simulink model "ev"  (R2021a)
settings: Solver=ode4  StartTime=0  StopTime=1082  FixedStep=sim_dt  RelTol=1e-3
model workspace (MAT data in the model file):
  T_eff_bp = [-270; -210; -150; -90; -30; 30; 90; 150; 210; 270]
  T_eff_bp_2 = [-270; -210; -150; -90; -30; 30; 90; 150; 210; 270]
  losses_table = [108927.107777 7820.2782368 7820.17609997 7820.2782368 7820.2782368 7820.2782368 7820.2782368 7820.26172359 7820.2782368 9345.38006027 108927.107777 7820.2782368 ... (100 elements, 10x10)]
  losses_table_2 = [108927.107777 7820.2782368 7820.17609997 7820.2782368 7820.2782368 7820.2782368 7820.2782368 7820.26172359 7820.2782368 9345.38006027 108927.107777 7820.2782368 ... (100 elements, 10x10)]
  w_eff_bp = [0; 888.888888889; 1777.77777778; 2666.66666667; 3555.55555556; 4444.44444444; 5333.33333333; 6222.22222222; 7111.11111111; 8000]
  w_eff_bp_2 = [0; 888.888888889; 1777.77777778; 2666.66666667; 3555.55555556; 4444.44444444; 5333.33333333; 6222.22222222; 7111.11111111; 8000]
undefined symbols (not defined in the file): Af, alpha, Bt, C, C_fa, C_free, C_sa_bat, C_sa_uc, Cd, Cmax, Continuous, Crr, DoD, effi, etaFD, etaG, FD, G, gear, Iucmax, m, M1m, M2m, Max, npar, npar_free, npara, nparf, nparfa, nparsa_bat, nparsa_UC, nser, nser_free, nserfa, nsersa_bat, nsersa_UC, Qbat, regenmax, Ri_BP, RL, ro, Rsc, Rsc_A, Rsc_F, Rsc_sa_bat, Rsc_sa_uc, rw, sim_dt, SOC_BP, SoCbatmax, SoCbatmin, SoCucmax, SoCucmin, speed, torque, VinBat, Voc_BP, Vuc, Vuc_fa, Vuc_free ... (+2)
libraries: autolibshared x41, simulink x26, autolibdcdc x13, autolibdatasheetbattery x7, autolibmappedmotor x6, fl_lib x3, nesl_utility x3, spsSupercapacitorLib x3, pid_lib x1
(part 9 of 18)

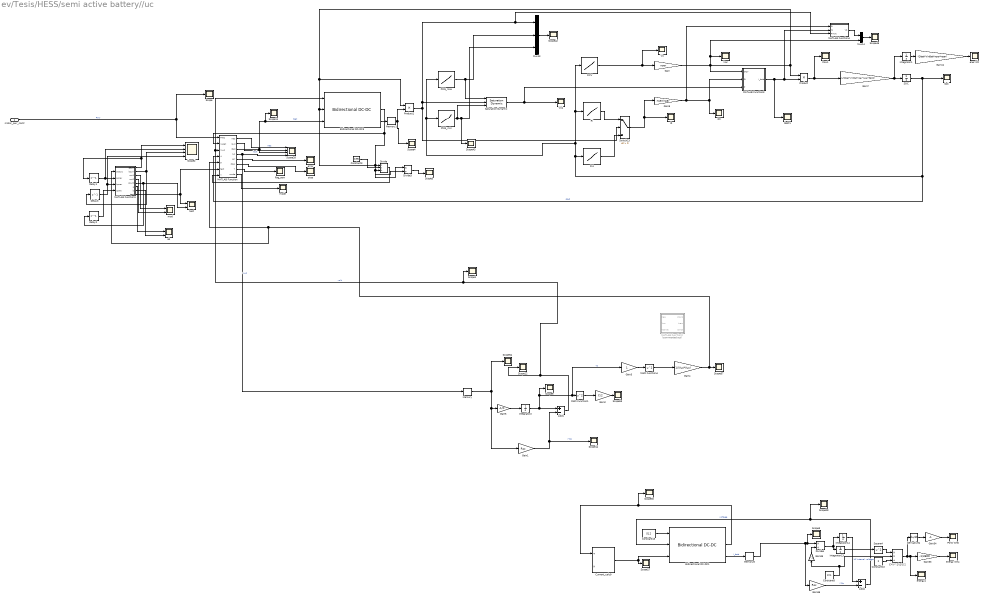
== system ev/Tesis/HESS/semi active battery//uc ==
  motor_pwr_contr : Inport
  Add1 : Sum  Inputs=+-
  Add4 : Sum  Inputs=+-
  Bidirectional DC-DC1 : autolibdcdc/Bidirectional DC-DC  Tc=1/1000  Vinit=51.2  Plimit=100000  param_loss=Single efficiency measurement  eff=95  v_loss_bp=[0 200 400 600 800 1000]  i_loss_bp=[0 25 50 75 100]  losses_table=[100 100 100 100 100;100 150 200 250 300;100 200 300 400 500;100 250 400 550 700;100 300 500 700 900;100 350 600 850 1100]  v_eff_bp=[200 400 600 800 1000]  i_eff_bp=[25 50 75 100]  efficiency_table=[96.2 98.1 98.7 99;98.1 99 99.4 99.5;98.7 99.4 99.6 99.7;99 99.5 99.7 99.8;99.2 99.6 99.7 99.8]  x_v_bp=[-1000 -800 -600 -400 -200 200 400 600 800 1000]  x_i_bp=[-100 -75 -50 -25 25 50 75 100]  x_losses_mat=[200.400801603196 225.67703109328 200.803212851408 201.612903225806 199.999999999997 200 225 200;160.320641282556 180.541624874624 201.005025125625 202.020202020203 200 200 180 160;180.541624874624 180.722891566267 181.086519114686 197.568389057748 194.999999999999 179.999999999997 180 180;201.005025125625 181.086519114686 202.020202020203 193.67991845056 190 200 179.999999999997 200;202.020202020203 197.568389057748 193.67991845056 197.505197505197 190 190 194.999999999999 200;200 194.999999999999 190 190 197.505197505197 193.67991845056 197.568389057748 202.020202020203;200 179.999999999997 200 190 193.67991845056 202.020202020203 181.086519114686 201.005025125625;180 180 179.999999999997 194.999999999999 197.568389057748 181.086519114686 180.722891566267 180.541624874624;160 180 200 200 202.020202020203 201.005025125625 180.541624874624 160.320641282556;200 225 200 199.999999999997 201.612903225806 200.803212851408 225.67703109328 200.400801603196]  RefBlkName='autolibdcdc/Bidirectional DC-DC'
      settings: SourceProductBaseCode=PW
  Bidirectional DC-DC3 : autolibdcdc/Bidirectional DC-DC  Tc=1/1000  Vinit=48  Plimit=100000  param_loss=Single efficiency measurement  eff=95  v_loss_bp=[0 200 400 600 800 1000]  i_loss_bp=[0 25 50 75 100]  losses_table=[100 100 100 100 100;100 150 200 250 300;100 200 300 400 500;100 250 400 550 700;100 300 500 700 900;100 350 600 850 1100]  v_eff_bp=[200 400 600 800 1000]  i_eff_bp=[25 50 75 100]  efficiency_table=[96.2 98.1 98.7 99;98.1 99 99.4 99.5;98.7 99.4 99.6 99.7;99 99.5 99.7 99.8;99.2 99.6 99.7 99.8]  x_v_bp=[-1000 -800 -600 -400 -200 200 400 600 800 1000]  x_i_bp=[-100 -75 -50 -25 25 50 75 100]  x_losses_mat=[200.400801603196 225.67703109328 200.803212851408 201.612903225806 199.999999999997 200 225 200;160.320641282556 180.541624874624 201.005025125625 202.020202020203 200 200 180 160;180.541624874624 180.722891566267 181.086519114686 197.568389057748 194.999999999999 179.999999999997 180 180;201.005025125625 181.086519114686 202.020202020203 193.67991845056 190 200 179.999999999997 200;202.020202020203 197.568389057748 193.67991845056 197.505197505197 190 190 194.999999999999 200;200 194.999999999999 190 190 197.505197505197 193.67991845056 197.568389057748 202.020202020203;200 179.999999999997 200 190 193.67991845056 202.020202020203 181.086519114686 201.005025125625;180 180 179.999999999997 194.999999999999 197.568389057748 181.086519114686 180.722891566267 180.541624874624;160 180 200 200 202.020202020203 201.005025125625 180.541624874624 160.320641282556;200 225 200 199.999999999997 201.612903225806 200.803212851408 225.67703109328 200.400801603196]  RefBlkName='autolibdcdc/Bidirectional DC-DC'
      settings: SourceProductBaseCode=PW
  C*(V^2)/2(1)2 : Product  Inputs=**/
  Constant10 : Constant  Value=2
  Constant13 : Constant  Value=51.2
  Constant3 : Constant  Value=0.95
  Constant8 : Constant  Value=C*1
  Current_calc9 : Product  Inputs=/*
  Delay1 : Delay  DelayLength=1  InitialCondition=1
  Delay2 : Delay  DelayLength=1  InitialCondition=1
  Delay3 : Delay  DelayLength=1  InitialCondition=1
  Derivative4 : Derivative
  Divide : Product  Inputs=**/
  Divide3 : Product  Inputs=*/
  Divide4 : Product  Inputs=*/
  Gain : Gain  Gain=nser
  Gain1 : Gain  Gain=Rsc
  Gain11 : Gain  Gain=(Qbat*VinBat*nser*npar)
  Gain2 : Gain  Gain=C/2
  Gain3 : Gain
  Gain33 : Gain  Gain=-1/3600
  Gain34 : Gain  Gain=-1
  Gain35 : Gain  Gain=-1
  Gain36 : Gain  Gain=Rsc
  Gain4 : Gain  Gain=1/(Vuc*Vuc)
  Gain5 : Gain  Gain=-1/C
  Gain6 : Gain  Gain=nser/npar
  Gain7 : Gain  Gain=1/(Qbat*VinBat*nser*npar*3600)
  Ibatt1 : Scope
  Integrator1 : Integrator
  Integrator13 : Integrator
  Integrator14 : Integrator  InitialCondition=Vuc*1
  Integrator2 : Integrator  InitialCondition=48  UpperSaturationLimit=Vuc  LowerSaturationLimit=Vuc*0
  MATLAB Function : MATLAB Function  TreatAsAtomicUnit=on
  MATLAB Function1 : MATLAB Function  TreatAsAtomicUnit=on
  MATLAB Function2 : MATLAB Function  Commented=on  TreatAsAtomicUnit=on
  MATLAB Function3 : MATLAB Function  TreatAsAtomicUnit=on
  MATLAB Function4 : MATLAB Function  TreatAsAtomicUnit=on
  Math Function1 : Math  Operator=square  SaturateOnIntegerOverflow=on
  Math Function4 : Math  Operator=square  SaturateOnIntegerOverflow=on
  Memory : Memory
  Memory1 : Memory
  Memory8 : Memory
  Mux13 : Mux  Inputs=3
  Mux14 : Mux  Inputs=2
  OCV : Lookup_n-D  NumberOfTableDimensions=1  BreakpointsForDimension1=SOC_BP  Table=Voc_BP  InternalRulePriority=Speed  RndMeth=Simplest  InputSameDT=on
  PMG_max : Lookup_n-D  NumberOfTableDimensions=1  BreakpointsForDimension1=SOC_BP  Table=Voc_BP*nser*3*50*npar  InternalRulePriority=Speed  RndMeth=Simplest  InputSameDT=on
  PMG_min : Lookup_n-D  NumberOfTableDimensions=1  BreakpointsForDimension1=SOC_BP  Table=-Voc_BP*nser*3*50*npar  InternalRulePriority=Speed  RndMeth=Simplest  InputSameDT=on
  POW Wh5 : Scope
  Pow1 : Scope
  Product : Product
  Product1 : Product
  Ri : Lookup_n-D  NumberOfTableDimensions=1  BreakpointsForDimension1=SOC_BP  Table=Ri_BP  InternalRulePriority=Speed  RndMeth=Simplest  InputSameDT=on
  Ri4 : Lookup_n-D  NumberOfTableDimensions=1  BreakpointsForDimension1=SOC_BP  Table=Ri_BP  InternalRulePriority=Speed  RndMeth=Simplest  InputSameDT=on
  SOC : Integrator  InitialCondition=(1-DoD)
  Saturation Dynamic : simulink/Discontinuities/Saturation Dynamic  OutMin=[]  OutMax=[]  OutDataTypeStr=Inherit: Same as second input  OutDataType=fixdt(1, 16)  OutScaling=2^-10  DoSatur=off
  Scope{,1,3..5,9,11..12,14,27,29..30,42..43,45,53..54,57} (18 alike) : Scope
  Scope2 : Scope  NumInputPorts=4
  Scope28 : Scope  NumInputPorts=4
  SoC : Scope
  Square4 : Math  Operator=square  SaturateOnIntegerOverflow=on
  Switch13 : Switch  Criteria=u2 > Threshold
  Vo : Scope
  Vo1 : Scope
  Voc : Scope
  ab : Scope  NumInputPorts=2
  ener Wh : Scope
  energy Wh4 : Scope
  energy4 : Scope
  error : Scope
  flag_pow : Scope
  iR : Scope
  iRt : Scope
  mod : Scope  NumInputPorts=2
  mode : Scope
  stop : Scope
  test : Scope  NumInputPorts=2
  wires:
  motor_pwr_contr/1 -> Scope/1, MATLAB Function/1(Preq)  "Pow"
  MATLAB Function/3(Ibat) -> Scope11/1, Bidirectional DC-DC3/3, Scope28/3  "Ibat"
  MATLAB Function1/1(acurr) -> Delay1/1, Scope2/1
  MATLAB Function1/2(bcurr) -> Delay3/1, Scope2/3
  MATLAB Function/2(Iout) -> Scope28/2  "Iout"
  MATLAB Function/1(Ireq) -> Scope28/1  "Ireq"
  MATLAB Function/5(err) -> error/1
  MATLAB Function/6(stop) -> stop/1
  MATLAB Function/7(flagpow) -> flag_pow/1
  MATLAB Function/8(mode) -> mode/1
  MATLAB Function1/3(mo1) -> mod/1
  Delay1/1 -> Scope2/2, MATLAB Function1/2(aprev)
  Delay3/1 -> Scope2/4, MATLAB Function1/3(bprev)
  MATLAB Function1/5(count) -> test/2, Delay2/1
  MATLAB Function1/4(mo2) -> mod/2
  Delay2/1 -> MATLAB Function1/4(cprev)
  MATLAB Function1/6(a) -> ab/1
  MATLAB Function1/7(b) -> ab/2
  MATLAB Function1/8(test) -> test/1, MATLAB Function/6(test)
  Gain1/1 -> Add1/2, Scope14/1  "i*Rs"
  Gain2/1 -> Scope53/1
  Math Function4/1 -> Gain4/1
  Gain4/1 -> MATLAB Function/5(SoCuc), MATLAB Function1/1(SoCuc), Scope57/1
  Math Function1/1 -> Gain2/1
  Gain5/1 -> Integrator2/1
  Gain3/1 -> Math Function4/1
  Add1/1 -> Scope12/1, Bidirectional DC-DC3/1, MATLAB Function/3(V_uc), Scope1/1  "volt"
  MATLAB Function/4(Iuc) -> Memory/1, Scope28/4  "I_uc"
  Integrator2/1 -> Scope9/1, Gain3/1, Math Function1/1, Add1/1  "Vc"
  Memory/1 -> Scope54/1, Gain1/1, Gain5/1
  PMG_max/1 -> Saturation Dynamic/1, Mux13/2
  MATLAB Function4/1(Vb) -> Mux14/1
  Saturation Dynamic/1 -> Vo1/1, MATLAB Function3/3(P)
  Integrator1/1 -> Gain11/1
  Gain6/1 -> MATLAB Function4/1(Ri), MATLAB Function3/2(Ri), iRt/1
  Mux14/1 -> Scope45/1
  Gain7/1 -> Integrator1/1, SOC/1
  SOC/1 -> PMG_max/1, PMG_min/1, OCV/1, Ri/1, Ri4/1, MATLAB Function/4(SoCbat), SoC/1  "SOC"
  Gain11/1 -> ener Wh/1
  Ri4/1 -> Switch13/3
  Ri/1 -> Switch13/1
  MATLAB Function3/1(I_batt) -> Ibatt1/1, MATLAB Function4/2(Ib), Product/2
  OCV/1 -> Vo/1, Gain/1
  Product/1 -> Pow1/1, Gain7/1
  Switch13/1 -> Gain6/1, iR/1
  Gain/1 -> Mux14/2, Voc/1, MATLAB Function3/1(OCV), Product/1, Product1/1, Divide3/2, Divide/1, Bidirectional DC-DC3/2
  PMG_min/1 -> Saturation Dynamic/3, Scope43/1, Mux13/3
  Mux13/1 -> Scope42/1
  Product1/1 -> Switch13/2, MATLAB Function4/3(Pmot), Mux13/1, Saturation Dynamic/2
  Bidirectional DC-DC3/2 -> Divide3/1, Divide/3, MATLAB Function/2(V_bat)
  Constant3/1 -> Divide/2
  Divide/1 -> MATLAB Function/7(convDCDC)
  Divide3/1 -> Scope5/1
  Bidirectional DC-DC3/3 -> Memory1/1
  Memory1/1 -> Scope4/1, Product1/2
  Memory8/1 -> Gain36/1, Divide4/1, Scope3/1
  Gain34/1 -> POW Wh5/1
  Divide4/1 -> Integrator13/1, Integrator14/1
  Add4/1 -> Bidirectional DC-DC1/2, Scope29/1  "voltage"
  Gain35/1 -> Divide4/2
  Gain36/1 -> Add4/2  "i*Rs"
  Bidirectional DC-DC1/2 -> Scope30/1, Current_calc9/1
  Current_calc9/1 -> Bidirectional DC-DC1/3, Scope27/1
  Gain33/1 -> energy Wh4/1
  Derivative4/1 -> Gain34/1
  Integrator14/1 -> Add4/1  "UC internal voltage"
  C*(V^2)/2(1)2/1 -> Derivative4/1, energy4/1, Gain33/1
  Square4/1 -> C*(V^2)/2(1)2/1
  Constant10/1 -> C*(V^2)/2(1)2/3
  Constant13/1 -> Bidirectional DC-DC1/1
  Integrator13/1 -> Square4/1
  Bidirectional DC-DC1/3 -> Memory8/1  "I_batt"
  ? -> Current_calc9/2  "Pow"
  Constant8/1 -> Gain35/1, C*(V^2)/2(1)2/2

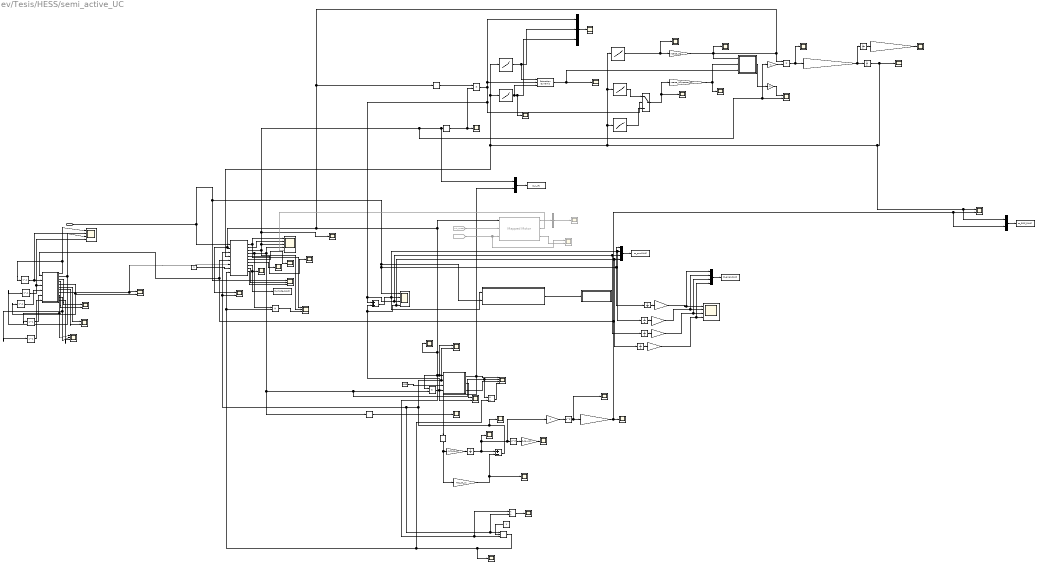
== system ev/Tesis/HESS/semi_active_UC ==
  motor_pwr_contr : Inport
  Add : Sum
  Add1 : Sum  Inputs=+-
  Bus Selector2 : BusSelector  Commented=on  OutputSignals=MechPwr
  Constant1 : Constant
  Constant5 : Constant  Value=0.95
  Constant6 : Constant
  Delay{4..8} (5 alike) : Delay  DelayLength=1  InitialCondition=0
  Divide1 : Product  Inputs=**/
  Divide3 : Product  Inputs=*/
  From1 : From  Commented=on  GotoTag=mtr_speed  TagVisibility=global
  From8 : From  Commented=on  GotoTag=mtr_trq_corr  TagVisibility=global
  Gain : Gain  Gain=nsersa_UC
  Gain1 : Gain  Gain=Rsc_sa_uc
  Gain{10,12..14} (4 alike) : Gain  Gain=1/(3600)
  Gain11 : Gain  Gain=(Qbat*VinBat*nsersa_UC*nparsa_UC)
  Gain2 : Gain  Gain=C_sa_uc/2
  Gain3 : Gain
  Gain4 : Gain  Gain=1/(Vuc_sa_uc*Vuc_sa_uc)
  Gain5 : Gain  Gain=-1/C_sa_uc
  Gain6 : Gain  Gain=nsersa_UC/nparsa_UC
  Gain7 : Gain  Gain=1/(Qbat*VinBat*nsersa_UC*nparsa_UC*3600)
  Gain8 : Gain  Gain=-1
  Gain9 : Gain  Gain=-1
  Ibatt1 : Scope  NumInputPorts=2
  Integrator{1,4..7} (5 alike) : Integrator
  Integrator2 : Integrator  InitialCondition=Vuc_sa_uc*0.95  UpperSaturationLimit=Vuc  LowerSaturationLimit=Vuc*0
  MATLAB Function : MATLAB Function  TreatAsAtomicUnit=on
  MATLAB Function2 : MATLAB Function  TreatAsAtomicUnit=on
  MATLAB Function3 : MATLAB Function  TreatAsAtomicUnit=on
  MATLAB Function4 : MATLAB Function  TreatAsAtomicUnit=on
  Mapped Motor3 : autolibmappedmotor/Mapped Motor  Commented=on  port_config=Speed  param_by=Tabulated torque-speed envelope  w_t=M1m'  T_t=-M2m'  torque_max=.1  power_max=30  Tc=0.02  param_loss=Tabulated loss data  eff=100  w_eff=375  T_eff=0.08  Piron=0  Pbase=0  w_eff_bp=w_eff_bp_2  T_eff_bp=T_eff_bp_2  Temp_eff_bp=[233.15 293.15 373.15]  losses_table=losses_table_2  losses_table_3d=cat(3,[1.49 1.67 2.21 3.10; 0.42 0.69 1.14 2.03; 0.06 0.24 0.78 1.68; 0.42 0.69 1.14 2.03; 1.49 1.67 2.21 3.10],[1.49 1.67 2.21 3.10; 0.42 0.69 1.14 2.03; 0.06 0.24 0.78 1.68; 0.42 0.69 1.14 2.03; 1.49 1.67 2.21 3.10],[1.49 1.67 2.21 3.10; 0.42 0.69 1.14 2.03; 0.06 0.24 0.78 1.68; 0.42 0.69 1.14 2.03; 1.49 1.67 2.21 3.10])  efficiency_table=loss_pow  efficiency_table_3d=cat(3,[95 95 95 95; 95 95 95 95; 95 95 95 95; 95 95 95 95; 95 95 95 95],[95 95 95 95; 95 95 95 95; 95 95 95 95; 95 95 95 95; 95 95 95 95],[95 95 95 95; 95 95 95 95; 95 95 95 95; 95 95 95 95; 95 95 95 95])  J=2.825e-002  b=0.2564  omega_o=0  T_t_extended=[-120.249620040167 -121.840837540031 -123.029026217228 -125.013569994029 -127.39293274711 -130.568650599794 -133.346564077512 -135.328122455626 -137.708231558378 -139.690536286164 -142.072138088259 -144.453739890354 -146.832356293763 -150.009566845791 -152.388929598871 -155.168335775932 -159.539705802529 -161.917575856267 -165.494083482603 -169.069098409597 -173.041917711556 -176.617678988221 -180.1904548662 -183.766216142865 -186.944173044564 -188.927970471693 -191.31031862346 -193.692666775227 -196.074268577322 -197.660261629485 -199.644059056614 -200.831501384139 -202.41152363893 -203.261615914889 -203.261615914889 -202.41152363893 -200.831501384139 -199.644059056614 -197.660261629485 -196.074268577322 -193.692666775227 -191.31031862346 -188.927970471693 -186.944173044564 -183.766216142865 -180.1904548662 -176.617678988221 -173.041917711556 -169.069098409597 -165.494083482603 -161.917575856267 -159.539705802529 -155.168335775932 -152.388929598871 -150.009566845791 -146.832356293763 -144.453739890354 -142.072138088259 -139.690536286164 -137.708231558378 -135.328122455626 -133.346564077512 -130.568650599794 -127.39293274711 -125.013569994029 -123.029026217228 -121.840837540031 -120.249620040167]  w_t_extended=[-899.138721392584 -895.216633185855 -885.411412669033 -874.625670100529 -858.937317273614 -842.268442395016 -826.580089568101 -811.872258792868 -797.164428017635 -783.437119294084 -770.690332622215 -757.943545950346 -741.274671071749 -726.566840296516 -710.8784874696 -697.151178746049 -680.482303867452 -662.832906937172 -649.105598213621 -633.417245386706 -616.748370508109 -602.040539732875 -583.410620750913 -568.702789975681 -554.975481252129 -543.209216631943 -531.442952011757 -519.67668739157 -506.929900719701 -496.144158151197 -484.37789353101 -473.592150962506 -454.962231980544 -0.980522051682199 0.980522051682199 454.962231980544 473.592150962506 484.37789353101 496.144158151197 506.929900719701 519.67668739157 531.442952011757 543.209216631943 554.975481252129 568.702789975681 583.410620750913 602.040539732875 616.748370508109 633.417245386706 649.105598213621 662.832906937172 680.482303867452 697.151178746049 710.8784874696 726.566840296516 741.274671071749 757.943545950346 770.690332622215 783.437119294084 797.164428017635 811.872258792868 826.580089568101 842.268442395016 858.937317273614 874.625670100529 885.411412669033 895.216633185855 899.138721392584]  KLossIron=0  KLossCopper=0  x_w_eff_vec=[-8000 -7111.11111111111 -6222.22222222222 -5333.33333333333 -4444.44444444444 -3555.55555555556 -2666.66666666667 -1777.77777777778 -888.888888888889 0 888.888888888889 1777.77777777778 2666.66666666667 3555.55555555556 4444.44444444444 5333.33333333333 6222.22222222222 7111.11111111111 8000]  x_T_eff_vec=[-270;-210;-150;-90;-30;30;90;150;210;270]  x_tmp_eff_vec=[-0.09 -0.06 -0.03 0 0.03 0.06 0.09]  x_losses_mat=[9345.3800602724 9345.3800602725 9345.3800602725 9345.38006027247 9345.38006027243 9345.38006027236 9345.38006027226 9345.38006027247 9345.38006027236 9345.3800602725;7820.27823680138 7820.27823680138 7820.27823680138 7820.27823680138 7820.27823680138 7820.27823680138 7820.27823680138 7820.27823680138 7820.27823680138 7820.27823680138;7820.26172358984 7820.26172358984 7820.26172358984 7820.26172358984 7820.26172358984 7820.26172358984 7820.26172358984 7820.26172358984 7820.26172358984 7820.26172358984;7820.27823680138 7820.27823680138 7820.27823680138 7820.27823680138 7820.27823680138 7820.27823680138 7820.27823680138 7820.27823680138 7820.27823680138 7820.27823680138;7820.27823680138 7820.27823680138 7820.27823680138 7820.27823680138 7820.27823680138 7820.27823680138 7820.27823680138 7820.27823680138 7820.27823680138 7820.27823680138;7820.27823680138 7820.27823680138 7820.27823680138 7820.27823680138 7820.27823680138 7820.27823680138 7820.27823680138 7820.27823680138 7820.27823680138 7820.27823680138;7820.27823680138 7820.27823680138 7820.27823680138 7820.27823680138 7820.27823680138 7820.27823680138 7820.27823680138 7820.27823680138 7820.27823680138 7820.27823680138;7820.17609997384 7820.17609997384 7820.17609997384 7820.17609997384 7820.17609997384 7820.17609997384 7820.17609997384 7820.17609997384 7820.17609997384 7820.17609997384;7820.27823680138 7820.27823680138 7820.27823680138 7820.27823680138 7820.27823680138 7820.27823680138 7820.27823680138 7820.27823680138 7820.27823680138 7820.27823680138;108927.107776947 108927.107776947 108927.107776947 108927.107776947 108927.107776947 108927.107776947 108927.107776947 108927.107776947 108927.107776947 108927.107776946;7820.27823680138 7820.27823680138 7820.27823680138 7820.27823680138 7820.27823680138 7820.27823680138 7820.27823680138 7820.27823680138 7820.27823680138 7820.27823680138;7820.17609997384 7820.17609997384 7820.17609997384 7820.17609997384 7820.17609997384 7820.17609997384 7820.17609997384 7820.17609997384 7820.17609997384 7820.17609997384;7820.27823680138 7820.27823680138 7820.27823680138 7820.27823680138 7820.27823680138 7820.27823680138 7820.27823680138 7820.27823680138 7820.27823680138 7820.27823680138;7820.27823680138 7820.27823680138 7820.27823680138 7820.27823680138 7820.27823680138 7820.27823680138 7820.27823680138 7820.27823680138 7820.27823680138 7820.27823680138;7820.27823680138 7820.27823680138 7820.27823680138 7820.27823680138 7820.27823680138 7820.27823680138 7820.27823680138 7820.27823680138 7820.27823680138 7820.27823680138;7820.27823680138 7820.27823680138 7820.27823680138 7820.27823680138 7820.27823680138 7820.27823680138 7820.27823680138 7820.27823680138 7820.27823680138 7820.27823680138;7820.26172358984 7820.26172358984 7820.26172358984 7820.26172358984 7820.26172358984 7820.26172358984 7820.26172358984 7820.26172358984 7820.26172358984 7820.26172358984;7820.27823680138 7820.27823680138 7820.27823680138 7820.27823680138 7820.27823680138 7820.27823680138 7820.27823680138 7820.27823680138 7820.27823680138 7820.27823680138;9345.3800602725 9345.38006027236 9345.38006027247 9345.38006027226 9345.38006027236 9345.38006027243 9345.38006027247 9345.3800602725 9345.3800602725 9345.3800602724]  x_losses_mat_3d=[37.8947368421052 25.2631578947368 12.6315789473684 0 12 24 36;18.9473684210526 12.6315789473684 6.3157894736842 0 5.99999999999999 12 18;0 0 0 0 0 0 0;18 12 5.99999999999999 0 6.3157894736842 12.6315789473684 18.9473684210526;36 24 12 0 12.6315789473684 25.2631578947368 37.8947368421052]  CalLossMapData={'BaseCageProjectFileName','CagePrj_1.cag';'BaseMbcProjectFileName','MbcPrj_1.mat';'TaskName','Calibrate Motor Loss Map';'ChildTasks',{{'DataName','MappedMotor-Loss : MappedMotor-Loss';'TaskName','Import Loss Data'},{'TaskName','Generate Response Models'},{'TaskName','Generate Calibration'},{'TaskName','Update Block Parameters'}}}  CalLossWithTempMapData={}  aMode=1  RefBlkName='autolibmappedmotor/Mapped Motor'
      settings: SourceProductBaseCode=PW,DR,MT,UV,VE
  Math Function1 : Math  Operator=square  SaturateOnIntegerOverflow=on
  Math Function4 : Math  Operator=square  SaturateOnIntegerOverflow=on
  Memory{,1..3} (4 alike) : Memory
  Mux1 : Mux
  Mux13 : Mux  Inputs=3
  Mux2 : Mux  Inputs=2
  Mux3 : Mux  Inputs=2
  Mux4 : Mux
  OCV : Lookup_n-D  NumberOfTableDimensions=1  BreakpointsForDimension1=SOC_BP  Table=Voc_BP  InternalRulePriority=Speed  RndMeth=Simplest  InputSameDT=on
  P : Scope
  PMG_max : Lookup_n-D  NumberOfTableDimensions=1  BreakpointsForDimension1=SOC_BP  Table=Voc_BP*nsersa_UC*Cmax*Qbat*nparsa_UC  InternalRulePriority=Speed  RndMeth=Simplest  InputSameDT=on
  PMG_min : Lookup_n-D  NumberOfTableDimensions=1  BreakpointsForDimension1=SOC_BP  Table=-Voc_BP*nsersa_UC*Cmax*Qbat*nparsa_UC  InternalRulePriority=Speed  RndMeth=Simplest  InputSameDT=on
  Pow1 : Scope
  Product{,1..3} (4 alike) : Product
  Product4 : Product  Inputs=*/
  Ri : Lookup_n-D  NumberOfTableDimensions=1  BreakpointsForDimension1=SOC_BP  Table=Ri_BP  InternalRulePriority=Speed  RndMeth=Simplest  InputSameDT=on
  Ri4 : Lookup_n-D  NumberOfTableDimensions=1  BreakpointsForDimension1=SOC_BP  Table=Ri_BP  InternalRulePriority=Speed  RndMeth=Simplest  InputSameDT=on
  SOC : Integrator  InitialCondition=(1-DoD)
  Saturation Dynamic : simulink/Discontinuities/Saturation Dynamic  OutMin=[]  OutMax=[]  OutDataTypeStr=Inherit: Same as second input  OutDataType=fixdt(1, 16)  OutScaling=2^-10  DoSatur=off
  Scope{1,4,9,11..12,14..17,42..43,53..54,57} (14 alike) : Scope
  Scope10 : Scope  NumInputPorts=4
  Scope{2,5,7,13} (4 alike) : Scope  NumInputPorts=2
  Scope19 : Scope  Commented=on
  Scope28 : Scope  NumInputPorts=5
  Scope3 : Scope  NumInputPorts=4
  Scope55 : Scope  NumInputPorts=3
  Scope6 : Scope  NumInputPorts=4
  Scope8 : Scope  Commented=on  NumInputPorts=2
  SoC : Scope
  Subsystem : Subsystem
  Switch13 : Switch  Criteria=u2 > Threshold
  To Workspace : ToWorkspace  VariableName=zz_powSAUC  SaveFormat=Structure With Time  SampleTime=-1
  To Workspace1 : ToWorkspace  VariableName=zz_SOC_SAUC  SaveFormat=Structure With Time  SampleTime=-1
  To Workspace2 : ToWorkspace  VariableName=zz_mode_SAUC  SaveFormat=Structure With Time  SampleTime=-1
  To Workspace3 : ToWorkspace  VariableName=zz_ener_SAUC  SaveFormat=Structure With Time  SampleTime=-1
  To Workspace4 : ToWorkspace  VariableName=zz_I_UC  SaveFormat=Structure With Time  SampleTime=-1
  Vo : Scope
  Voc : Scope
  ab1 : Scope  NumInputPorts=2
  ab2 : Scope  NumInputPorts=3
  ener Wh : Scope
  ener Wh2 : Scope  NumInputPorts=4
  error : Scope
  error1 : Scope  NumInputPorts=3
  flag_pow : Scope
  iR : Scope
  iRt : Scope
  mod1 : Scope  NumInputPorts=2
  mode : Scope
  stop : Scope
  test1 : Scope  NumInputPorts=2
  vehicle dynamics : Subsystem
  wires:
  motor_pwr_contr/1 -> Subsystem/2(motor_pwr_contr), Scope10/1, Integrator4/1, Mux1/1, Scope55/1, MATLAB Function/1(Preq)  "Pow"
  MATLAB Function/3(Ibat) -> error1/2, Gain8/1, Ibatt1/2, Mux3/1, Memory1/1, Scope11/1, Scope28/3  "Ibat"
  MATLAB Function/2(Iout) -> Scope28/2  "Iout"
  MATLAB Function/5(err) -> error/1
  MATLAB Function/6(stop) -> stop/1
  MATLAB Function/7(flagpow) -> flag_pow/1
  MATLAB Function/8(mode) -> To Workspace2/1, mode/1
  Gain1/1 -> Add1/2, Scope14/1  "i*Rs"
  Gain2/1 -> Scope53/1
  Math Function1/1 -> Gain2/1
  Gain5/1 -> Integrator2/1
  Gain3/1 -> Math Function4/1
  MATLAB Function/4(Iuc) -> Product3/1, Memory/1, Product2/2, Product4/1, Scope6/2, Scope28/4  "Iuc"
  Integrator2/1 -> Scope9/1, Gain3/1, Math Function1/1, Add1/1  "Vc"
  MATLAB Function3/1(Id) -> Mux3/2, Scope6/1, Memory3/1
  Memory/1 -> Scope54/1
  Constant5/1 -> MATLAB Function3/3(eff)
  MATLAB Function3/2(Pd) -> Scope5/1
  MATLAB Function3/3(Io) -> Scope6/3
  PMG_max/1 -> Saturation Dynamic/1, Mux13/2
  Gain7/1 -> Integrator1/1, SOC/1
  PMG_min/1 -> Saturation Dynamic/3, Scope43/1, Mux13/3
  Product/1 -> Pow1/1, Gain7/1
  Saturation Dynamic/1 -> P/1, MATLAB Function2/3(P)
  Gain11/1 -> ener Wh/1
  Switch13/1 -> Gain6/1, iR/1
  Integrator1/1 -> Gain11/1
  OCV/1 -> Vo/1, Gain/1
  Ri/1 -> Switch13/1
  Mux13/1 -> Scope42/1
  Ri4/1 -> Switch13/3
  SOC/1 -> Mux2/1, Scope13/1, PMG_max/1, PMG_min/1, MATLAB Function/4(SoCbat), Ri4/1, OCV/1, Ri/1, SoC/1  "SOC bat"
  Gain6/1 -> MATLAB Function2/2(Ri), iRt/1
  MATLAB Function2/1(I_batt) -> Gain9/1
  Gain8/1 -> Product/2
  Gain9/1 -> Ibatt1/1
  Memory1/1 -> Product1/2, Scope15/1
  Memory2/1 -> Product1/1
  Add1/1 -> Divide3/2, Divide1/1, MATLAB Function/3(V_uc), Scope2/2, Scope7/2, MATLAB Function3/2(Vd), Scope12/1
  Gain/1 -> Voc/1, MATLAB Function2/1(OCV), Product/1, Memory2/1, Mapped Motor3/1, Scope7/1, MATLAB Function3/1(Vo), Divide3/1, Divide1/3, Product2/1, Scope1/1, MATLAB Function/2(V_bat), Scope2/1  "volt"
  Constant6/1 -> Divide1/2
  Divide3/1 -> Scope17/1
  Divide1/1 -> Product4/2, Product3/2, MATLAB Function/8(conDCDC), Scope16/1
  MATLAB Function/1(Ireq) -> Scope28/1, error1/1  "Ireq"
  Constant1/1 -> MATLAB Function/7(convDCDC)
  MATLAB Function4/11(countc) -> ab2/3
  Delay8/1 -> MATLAB Function4/6(cprevb)
  MATLAB Function4/10(countb) -> ab2/2, Delay8/1
  MATLAB Function4/9(counta) -> ab2/1, Delay7/1
  Delay7/1 -> MATLAB Function4/5(cpreva)
  MATLAB Function4/6(a) -> ab1/1
  MATLAB Function4/7(b) -> ab1/2
  MATLAB Function4/5(count) -> Delay5/1, test1/2
  MATLAB Function4/8(test) -> MATLAB Function/6(test), test1/1
  MATLAB Function4/4(mo2) -> mod1/2
  Delay4/1 -> Scope3/2, MATLAB Function4/2(aprev)
  MATLAB Function4/1(acurr) -> Delay4/1, Scope3/1
  Gain4/1 -> Scope57/1, MATLAB Function4/1(SoCuc), MATLAB Function/5(SoCuc), Mux2/2, Scope13/2  "SOC UC"
  Delay5/1 -> MATLAB Function4/4(cprev)
  Delay6/1 -> Scope3/4, MATLAB Function4/3(bprev)
  MATLAB Function4/2(bcurr) -> Scope3/3, Delay6/1
  MATLAB Function4/3(mo1) -> mod1/1
  Math Function4/1 -> Scope4/1, Gain4/1  "SOC UC"
  From8/1 -> Scope8/1, Mapped Motor3/3
  Mapped Motor3/3 -> Scope8/2
  Mapped Motor3/2 -> Scope28/5
  Bus Selector2/1 -> Scope19/1  "<MechPwr>"
  Mapped Motor3/1 -> Bus Selector2/1
  From1/1 -> Mapped Motor3/2
  Subsystem/1(Out1) -> vehicle dynamics/1("Force_FA ")
  Add/1 -> Integrator5/1, Mux1/2, Scope10/2, Subsystem/1(In1)
  Product1/1 -> Integrator6/1, Mux1/3, Scope10/3, Add/1, Switch13/2, Mux13/1, Saturation Dynamic/2
  Product2/1 -> Integrator7/1, Mux1/4, Scope10/4, Add/2, Scope5/2, MATLAB Function3/4(Po)
  Mux2/1 -> To Workspace1/1
  Mux1/1 -> To Workspace/1
  Mux4/1 -> To Workspace3/1
  Gain13/1 -> Mux4/4, ener Wh2/4
  Gain12/1 -> Mux4/3, ener Wh2/3
  Gain14/1 -> Mux4/1, ener Wh2/1
  Gain10/1 -> Mux4/2, ener Wh2/2
  Integrator7/1 -> Gain13/1
  Integrator4/1 -> Gain14/1
  Integrator6/1 -> Gain12/1
  Integrator5/1 -> Gain10/1
  MATLAB Function/9(Pdispm) -> Scope55/2
  MATLAB Function/10(Pdispn) -> Scope55/3
  Product3/1 -> error1/3
  Product4/1 -> Scope6/4
  Memory3/1 -> Gain1/1, Gain5/1
  Mux3/1 -> To Workspace4/1

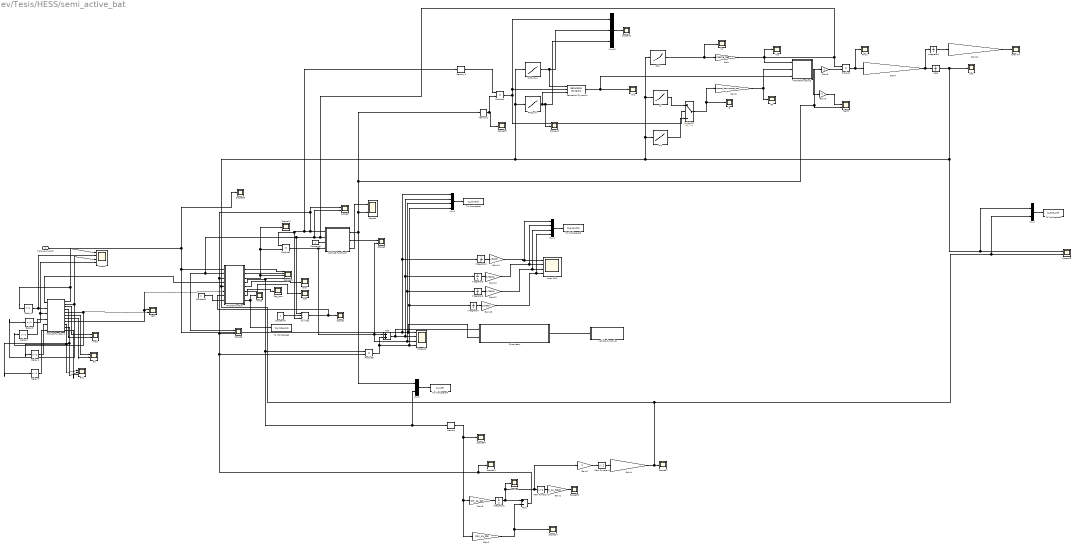
== system ev/Tesis/HESS/semi_active_bat ==
  motor_pwr_contr : Inport
  Add : Sum
  Add1 : Sum  Inputs=+-
  Constant1 : Constant
  Constant3 : Constant
  Constant4 : Constant
  Delay{1..5} (5 alike) : Delay  DelayLength=1  InitialCondition=0
  Divide1 : Product  Inputs=**/
  Gain : Gain  Gain=nsersa_bat
  Gain1 : Gain  Gain=Rsc_sa_bat
  Gain{10,12..14} (4 alike) : Gain  Gain=1/(3600)
  Gain11 : Gain  Gain=(Qbat*VinBat*nsersa_bat*nparsa_bat)
  Gain2 : Gain  Gain=C_sa_bat/2
  Gain3 : Gain
  Gain4 : Gain  Gain=1/(Vuc_sa_bat*Vuc_sa_bat)
  Gain5 : Gain  Gain=-1/C_sa_bat
  Gain6 : Gain  Gain=nsersa_bat/nparsa_bat
  Gain7 : Gain  Gain=1/(Qbat*VinBat*nsersa_bat*nparsa_bat*3600)
  Gain8 : Gain  Gain=-1
  Gain9 : Gain  Gain=-1
  Ibatt1 : Scope  NumInputPorts=2
  Integrator{1,4..7} (5 alike) : Integrator
  Integrator2 : Integrator  InitialCondition=Vuc_sa_bat*0.95  UpperSaturationLimit=Vuc  LowerSaturationLimit=Vuc*0
  MATLAB Function : MATLAB Function  TreatAsAtomicUnit=on
  MATLAB Function1 : MATLAB Function  TreatAsAtomicUnit=on
  MATLAB Function2 : MATLAB Function  TreatAsAtomicUnit=on
  MATLAB Function5 : MATLAB Function  TreatAsAtomicUnit=on
  Math Function1 : Math  Operator=square  SaturateOnIntegerOverflow=on
  Math Function4 : Math  Operator=square  SaturateOnIntegerOverflow=on
  Memory : Memory
  Memory1 : Memory
  Memory2 : Memory
  Mux1 : Mux
  Mux13 : Mux  Inputs=3
  Mux2 : Mux  Inputs=2
  Mux3 : Mux  Inputs=2
  Mux4 : Mux
  OCV : Lookup_n-D  NumberOfTableDimensions=1  BreakpointsForDimension1=SOC_BP  Table=Voc_BP  InternalRulePriority=Speed  RndMeth=Simplest  InputSameDT=on
  PMG_max : Lookup_n-D  NumberOfTableDimensions=1  BreakpointsForDimension1=SOC_BP  Table=Voc_BP*nsersa_bat*Cmax*Qbat*nparsa_bat  InternalRulePriority=Speed  RndMeth=Simplest  InputSameDT=on
  PMG_min : Lookup_n-D  NumberOfTableDimensions=1  BreakpointsForDimension1=SOC_BP  Table=-Voc_BP*nsersa_bat*Cmax*Qbat*nparsa_bat  InternalRulePriority=Speed  RndMeth=Simplest  InputSameDT=on
  Pow1 : Scope
  Product{,1..3} (4 alike) : Product
  Ri : Lookup_n-D  NumberOfTableDimensions=1  BreakpointsForDimension1=SOC_BP  Table=Ri_BP  InternalRulePriority=Speed  RndMeth=Simplest  InputSameDT=on
  Ri4 : Lookup_n-D  NumberOfTableDimensions=1  BreakpointsForDimension1=SOC_BP  Table=Ri_BP  InternalRulePriority=Speed  RndMeth=Simplest  InputSameDT=on
  SOC : Integrator  InitialCondition=(1-DoD)
  Saturation Dynamic : simulink/Discontinuities/Saturation Dynamic  OutMin=[]  OutMax=[]  OutDataTypeStr=Inherit: Same as second input  OutDataType=fixdt(1, 16)  OutScaling=2^-10  DoSatur=off
  Scope{1,9,11..12,14..15,42..43,53..55,57} (12 alike) : Scope
  Scope10 : Scope  NumInputPorts=4
  Scope{3..5,8,13} (5 alike) : Scope  NumInputPorts=2
  Scope2 : Scope  NumInputPorts=4
  Scope28 : Scope  NumInputPorts=4
  SoC : Scope
  Subsystem : Subsystem
  Switch13 : Switch  Criteria=u2 > Threshold
  To Workspace : ToWorkspace  VariableName=zz_powSAb  SaveFormat=Structure With Time  SampleTime=-1
  To Workspace1 : ToWorkspace  VariableName=zz_SOC_SAb  SaveFormat=Structure With Time  SampleTime=-1
  To Workspace2 : ToWorkspace  VariableName=zz_mode_SAb  SaveFormat=Structure With Time  SampleTime=-1
  To Workspace3 : ToWorkspace  VariableName=zz_ener_SAb  SaveFormat=Structure With Time  SampleTime=-1
  To Workspace4 : ToWorkspace  VariableName=zz_I_bat  SaveFormat=Structure With Time  SampleTime=-1
  Vo : Scope
  Vo1 : Scope
  Voc : Scope
  ab : Scope  NumInputPorts=2
  ab1 : Scope  NumInputPorts=3
  ener Wh : Scope
  ener Wh2 : Scope  NumInputPorts=4
  error : Scope
  flag_pow : Scope
  iR : Scope
  iRt : Scope
  mod : Scope  NumInputPorts=2
  mode : Scope
  stop : Scope
  test : Scope  NumInputPorts=2
  vehicle dynamics : Subsystem
  wires:
  motor_pwr_contr/1 -> Mux1/1, Integrator4/1, Subsystem/2(motor_pwr_contr), Scope10/1, MATLAB Function/1(Preq), Scope55/1  "Pow"
  MATLAB Function/3(Ibat) -> Scope11/1, Product2/2, Scope28/3  "I bat"
  MATLAB Function/2(Iout) -> Scope28/2  "Iout tot"
  MATLAB Function/5(err) -> error/1
  MATLAB Function/6(stop) -> stop/1
  MATLAB Function/7(flagpow) -> flag_pow/1
  MATLAB Function/8(mode) -> mode/1, To Workspace2/1
  Gain1/1 -> Add1/2, Scope14/1  "i*Rs"
  Gain2/1 -> Scope53/1
  Math Function4/1 -> Gain4/1
  Math Function1/1 -> Gain2/1
  Gain5/1 -> Integrator2/1
  Gain3/1 -> Math Function4/1
  MATLAB Function/4(Iuc) -> Product3/1, Mux3/2, Memory/1, Scope28/4  "I uc"
  Integrator2/1 -> Scope9/1, Gain3/1, Math Function1/1, Add1/1  "Vc"
  Memory/1 -> Gain1/1, Gain5/1, Scope54/1
  Constant3/1 -> MATLAB Function5/3(eff)
  MATLAB Function5/2(Pd) -> Scope3/1
  Add/1 -> Subsystem/1(In1), Mux1/2, Integrator5/1, Scope10/2
  MATLAB Function5/1(Id) -> Mux3/1, Memory1/1, Gain8/1, Ibatt1/2, Scope4/2
  PMG_max/1 -> Saturation Dynamic/1, Mux13/2
  Gain7/1 -> Integrator1/1, SOC/1
  PMG_min/1 -> Saturation Dynamic/3, Scope43/1, Mux13/3
  Product/1 -> Pow1/1, Gain7/1
  Saturation Dynamic/1 -> Vo1/1, MATLAB Function2/3(P)
  Gain11/1 -> ener Wh/1
  Switch13/1 -> Gain6/1, iR/1
  Integrator1/1 -> Gain11/1
  OCV/1 -> Vo/1, Gain/1
  Ri/1 -> Switch13/1
  Mux13/1 -> Scope42/1
  Ri4/1 -> Switch13/3
  Product1/1 -> Switch13/2, Mux13/1, Saturation Dynamic/2
  Gain6/1 -> MATLAB Function2/2(Ri), iRt/1
  MATLAB Function5/3(Io) -> Scope4/1
  MATLAB Function2/1(I_batt) -> Gain9/1
  Gain8/1 -> Product/2
  Gain9/1 -> Ibatt1/1
  Memory1/1 -> Product1/2, Scope15/1
  Memory2/1 -> Product1/1
  Constant1/1 -> MATLAB Function/8(conDCDC)
  Constant4/1 -> Divide1/2
  Divide1/1 -> MATLAB Function/7(convDCDC), Scope1/1
  Gain/1 -> Voc/1, MATLAB Function2/1(OCV), Product/1, MATLAB Function/2(V_bat), Scope5/1, Divide1/1, Scope8/2, MATLAB Function5/2(Vd)
  MATLAB Function/1(Ireq) -> Scope28/1  "Ireq"
  Product2/1 -> Scope3/2, Mux1/3, Integrator6/1, Scope10/3, Add/1, MATLAB Function5/4(Po)
  MATLAB Function1/11(countc) -> ab1/3
  Delay5/1 -> MATLAB Function1/6(cprevb)
  MATLAB Function1/10(countb) -> ab1/2, Delay5/1
  MATLAB Function1/9(counta) -> ab1/1, Delay4/1
  Delay4/1 -> MATLAB Function1/5(cpreva)
  MATLAB Function1/6(a) -> ab/1
  MATLAB Function1/7(b) -> ab/2
  MATLAB Function1/5(count) -> Delay2/1, test/2
  MATLAB Function1/8(test) -> MATLAB Function/6(test), test/1
  MATLAB Function1/4(mo2) -> mod/2
  Delay1/1 -> Scope2/2, MATLAB Function1/2(aprev)
  MATLAB Function1/1(acurr) -> Delay1/1, Scope2/1
  Delay2/1 -> MATLAB Function1/4(cprev)
  Delay3/1 -> Scope2/4, MATLAB Function1/3(bprev)
  MATLAB Function1/2(bcurr) -> Scope2/3, Delay3/1
  MATLAB Function1/3(mo1) -> mod/1
  Product3/1 -> Mux1/4, Integrator7/1, Scope10/4, Add/2
  Add1/1 -> Product3/2, Memory2/1, Product2/1, Divide1/3, MATLAB Function5/1(Vo), Scope8/1, MATLAB Function/3(V_uc), Scope5/2, Scope12/1
  Subsystem/1(Out1) -> vehicle dynamics/1("Force_FA ")
  Mux1/1 -> To Workspace/1
  Mux2/1 -> To Workspace1/1
  Integrator7/1 -> Gain13/1
  Integrator5/1 -> Gain10/1
  Integrator6/1 -> Gain12/1
  Integrator4/1 -> Gain14/1
  Gain10/1 -> Mux4/2, ener Wh2/2
  Gain14/1 -> Mux4/1, ener Wh2/1
  Gain12/1 -> Mux4/3, ener Wh2/3
  Gain13/1 -> Mux4/4, ener Wh2/4
  Mux4/1 -> To Workspace3/1
  Gain4/1 -> Mux2/2, Scope13/2, MATLAB Function1/1(SoCuc), MATLAB Function/5(SoCuc), Scope57/1  "SOC UC"
  SOC/1 -> Mux2/1, Scope13/1, PMG_max/1, PMG_min/1, MATLAB Function/4(SoCbat), Ri4/1, OCV/1, Ri/1, SoC/1  "SOC bat"
  Mux3/1 -> To Workspace4/1

== system ev/Tesis/Battery model/Subsystem/motor speed estimation ==
  vel_m/s : Inport
  Gain : Gain  Gain=1/(rw)
  Scope1 : Scope
  transmission : Product
  motor angular speed : Outport
  wires:
  transmission/1 -> motor angular speed/1, Scope1/1  "motor angular speed"
  [gear_ratio] -> transmission/2
  Gain/1 -> transmission/1  "wheel angular speed"
  vel_m/s/1 -> Gain/1

== system ev/Tesis/HESS/Free/Subsystem ==
  In1 : Inport
  motor_pwr_contr : Inport  Port=2
  1-D Lookup Table : Lookup_n-D  NumberOfTableDimensions=1  BreakpointsForDimension1=Continuous(:,1)  Table=Continuous(:,2)  InternalRulePriority=Speed  RndMeth=Simplest  InputSameDT=on
  1-D Lookup Table2 : Lookup_n-D  NumberOfTableDimensions=1  BreakpointsForDimension1=Continuous(:,1)  Table=-Continuous(:,2)  InternalRulePriority=Speed  RndMeth=Simplest  InputSameDT=on
  Constant : Constant  Value=0
  Constant1 : Constant
  Divide1 : Product  Inputs=**
  Divide2 : Product  Inputs=**
  Divide3 : Product  Inputs=*/
  Gain2 : Gain  Gain=30/pi
  Gain4 : Gain  Gain=0.95
  Gain5 : Gain  Gain=1/rw
  Gain6 : Gain  Gain=1/0.95
  Manual Switch : ManualSwitch  CurrentSetting=0
  Saturation Dynamic : simulink/Discontinuities/Saturation Dynamic  OutMin=[]  OutMax=[]  OutDataTypeStr=Inherit: Same as second input  OutDataType=fixdt(1, 16)  OutScaling=2^-10  DoSatur=off
  Scope : Scope
  Scope1 : Scope
  Switch : Switch  Criteria=u2 ~= 0
  Switch1 : Switch
  Switch2 : Switch  Criteria=u2 ~= 0
  motor speed estimation : Subsystem
  Out1 : Outport
  wires:
  motor_pwr_contr/1 -> Switch1/2
  Gain4/1 -> Divide1/1  "breaking torque"
  [gear_ratio] -> Divide1/2
  Divide1/1 -> Switch1/1
  Switch1/1 -> Gain5/1  "motor torque"
  Gain5/1 -> Out1/1  "FORCE"
  [gear_ratio] -> Divide2/2
  Gain6/1 -> Divide2/1  "motor_torque"
  Divide2/1 -> Switch1/3
  Divide3/1 -> Switch/1, Scope/1  "torque"
  In1/1 -> Divide3/1  "power"
  Gain2/1 -> 1-D Lookup Table2/1, 1-D Lookup Table/1
  1-D Lookup Table/1 -> Saturation Dynamic/1
  1-D Lookup Table2/1 -> Saturation Dynamic/3
  Saturation Dynamic/1 -> Gain4/1, Gain6/1
  Switch/1 -> Saturation Dynamic/2
  Constant/1 -> Switch/3
  motor speed estimation/1(motor angular speed) -> Manual Switch/2  "motor angular speed required"
  Manual Switch/1 -> Scope1/1, Gain2/1, Switch2/1, Switch2/2, Switch/2
  [mtr_speed] -> Manual Switch/1
  [Veh_real_pass] -> motor speed estimation/1(vel_m/s)
  Switch2/1 -> Divide3/2
  Constant1/1 -> Switch2/3
